simulink model "dynamic_plaque_model"  (R2021a)
settings: Solver=FixedStepAuto  StartTime=0.0  StopTime=10.0  RelTol=1e-3
values from neighbouring files (symbols this model uses):
  Fg_sphere = masseS*g    (= 0.07848)    [Constante_NL.m]
  Fg_total = masseTotal*g    (= 4.24773)    [Constante_NL.m]
  Jp = 1.347*10^-3    (= 0.001347)    [Constante_NL.m]
  masseTotal = masseP + sig*masseS    (= 0.433)    [Constante_NL.m]
  XA = +rABC    (= 0.0952)    [Constante_NL.m]
  XB = -rABC*sind(30)    [Constante_NL.m]
  XC = -rABC*sind(30)    [Constante_NL.m]
  YA = 0.0    (= 0)    [Constante_NL.m]
  YB = +rABC*cosd(30)    [Constante_NL.m]
  YC = -rABC*cosd(30)    [Constante_NL.m]
settings Model: Creator=dupa1607  LastModifiedBy=antho
settings SolverCC: AlgebraicLoopSolver=TrustRegion
settings DebuggingCC: SFMachineParentedDataDiag=warning

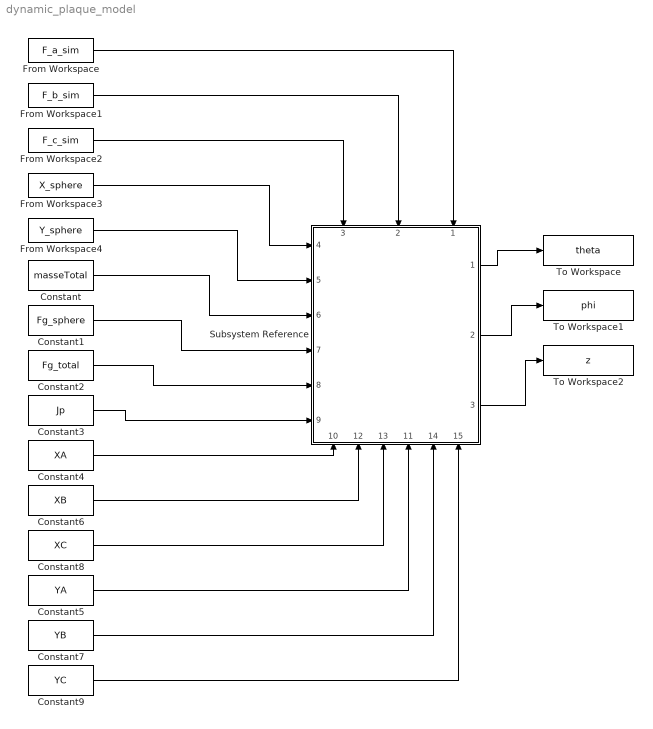
== system dynamic_plaque_model ==
  Constant : Constant  Value=masseTotal
  Constant1 : Constant  Value=Fg_sphere
  Constant2 : Constant  Value=Fg_total
  Constant3 : Constant  Value=Jp
  Constant4 : Constant  Value=XA
  Constant5 : Constant  Value=YA
  Constant6 : Constant  Value=XB
  Constant7 : Constant  Value=YB
  Constant8 : Constant  Value=XC
  Constant9 : Constant  Value=YC
  From Workspace : FromWorkspace  VariableName=F_a_sim
  From Workspace1 : FromWorkspace  VariableName=F_b_sim
  From Workspace2 : FromWorkspace  VariableName=F_c_sim
  From Workspace3 : FromWorkspace  VariableName=X_sphere
  From Workspace4 : FromWorkspace  VariableName=Y_sphere
  Subsystem Reference : Subsystem  ReferencedSubsystem=subsys_dynamic_plaque
      settings: PortSchema="{\"entries\":[{\"content\":{\"sides\":[{\"content\":{\"connectorIds\":[\"In4\",\"In5\",\"In6\",\"In7\",\"In8\",\"In9\"]},\"type\":\"ConnectorPlacement.EquallySpacedRectSide\",\"uuid\":\"ab2b7aea-a704-4e49-bcb9-ce0fc72e24a6\"},{\"content\":{\"connectorIds\":[\"Out1\",\"Out2\",\"Out3\"],\"side\":\"RIGHT\"},\"type\":\"ConnectorPlacement.EquallySpacedRectSide\",\"uuid\":\"ff8370ca-3f2d-4db7-87e6-1ea65707c64e\"},{\"content\":{\"connectorIds\":[\"In3\",\"In2\",\"In1\"],\"side\":\"TOP\"},\"type\":\"ConnectorPlacement.EquallySpacedRectSide\",\"uuid\":\"7d6a6474-0726-4322-82cf-c0c021e7caf1\"},{\"content\":{\"connectorIds\":[\"In10\",\"In12\",\"In13\",\"In11\",\"In14\",\"In15\"],\"side\":\"BOTTOM\"},\"type\":\"ConnectorPlacement.EquallySpacedRectSide\",\"uuid\":\"3e7879e2-18bf-4e3b-81d3-ac675b72e809\"}]},\"type\":\"ConnectorPlacement.EquallySpacedConnector\",\"uuid\":\"e2ea64f6-a590-4777-a4b3-11e2832a2548\"}],\"packageUris\":[\"http://schema.mathworks.com/mf0/Connector/R2020b\"],\"version\":\"1.0\"}"
  To Workspace : ToWorkspace  VariableName=theta  SaveFormat=Timeseries  SampleTime=-1
  To Workspace1 : ToWorkspace  VariableName=phi  SaveFormat=Timeseries  SampleTime=-1
  To Workspace2 : ToWorkspace  VariableName=z  SaveFormat=Timeseries  SampleTime=-1
  wires:
  From Workspace/1 -> Subsystem Reference/1
  From Workspace1/1 -> Subsystem Reference/2
  From Workspace2/1 -> Subsystem Reference/3
  Subsystem Reference/3 -> To Workspace2/1
  Subsystem Reference/2 -> To Workspace1/1
  Subsystem Reference/1 -> To Workspace/1
  From Workspace3/1 -> Subsystem Reference/4
  From Workspace4/1 -> Subsystem Reference/5
  Constant/1 -> Subsystem Reference/6
  Constant1/1 -> Subsystem Reference/7
  Constant2/1 -> Subsystem Reference/8
  Constant3/1 -> Subsystem Reference/9
  Constant4/1 -> Subsystem Reference/10
  Constant5/1 -> Subsystem Reference/11
  Constant6/1 -> Subsystem Reference/12
  Constant9/1 -> Subsystem Reference/15
  Constant8/1 -> Subsystem Reference/13
  Constant7/1 -> Subsystem Reference/14
